simulink model "AKZO_NOBEL"  (Simulink 8.0)
settings: Solver=ode15s  StartTime=0.0  StopTime=180.0  RelTol=1e-10
PreLoadFcn:
  | k1=18.7; k2=.58; k3=.09; k4=.42; K=34.4; klA=3.3; Ks=115.83; pCO2=.9; H=737;
settings Model: Creator=David  LastModifiedBy=David
settings DataIOCC: LimitDataPoints=off  SignalLoggingSaveFormat=ModelDataLogs
settings DebuggingCC: FcnCallInpInsideContextMsg=UseLocalSettings
settings GRTTargetCC: CombineOutputUpdateFcns=off  GRTInterface=on

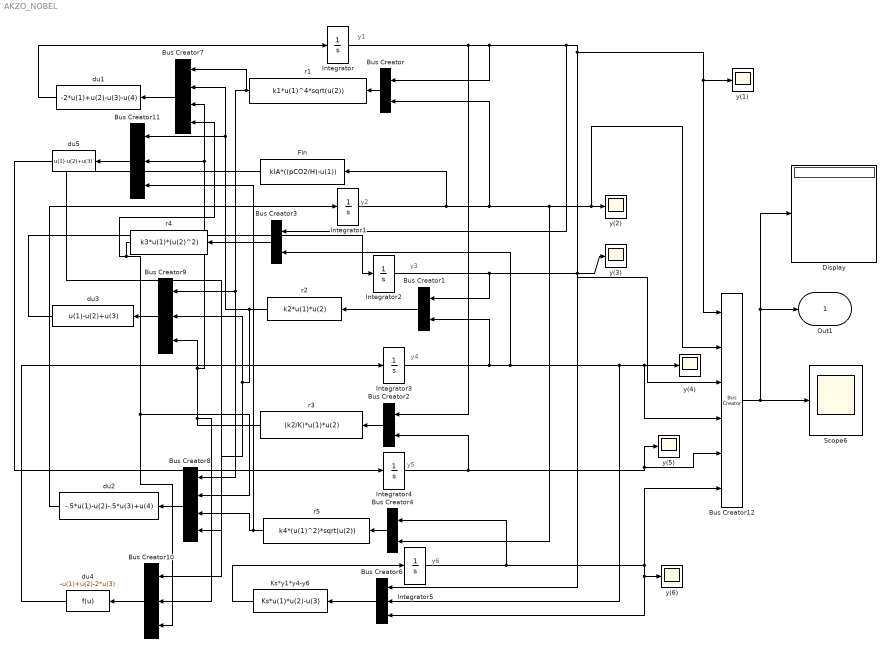
== system AKZO_NOBEL ==
  note: y1
  note: y2
  note: y3
  note: y4
  note: y5
  note: y6
  Bus Creator{,1..4} (5 alike) : BusCreator  Inputs=2
  Bus Creator{6,9..11} (4 alike) : BusCreator  Inputs=3
  Bus Creator12 : BusCreator  Inputs=6
  Bus Creator7 : BusCreator
  Bus Creator8 : BusCreator
  Display : Display
  Fin : Fcn  Expr=klA*((pCO2/H)-u(1))
  Integrator : Integrator  InitialCondition=.437
  Integrator1 : Integrator  InitialCondition=.00123
  Integrator2 : Integrator
  Integrator3 : Integrator  InitialCondition=.007
  Integrator4 : Integrator
  Integrator5 : Integrator  InitialCondition=115.83*.437*.007
  Ks*y1*y4-y6 : Fcn  Expr=Ks*u(1)*u(2)-u(3)
  Scope6 : Scope
      settings: SaveName=ScopeData6
  du1 : Fcn  Expr=-2*u(1)+u(2)-u(3)-u(4)
  du2 : Fcn  Expr=-.5*u(1)-u(2)-.5*u(3)+u(4)
  du3 : Fcn  Expr=u(1)-u(2)+u(3)
  du4 : Fcn  Expr=-u(1)+u(2)-2*u(3)
  du5 : Fcn  Expr=u(1)-u(2)+u(3)
  r1 : Fcn  Expr=k1*u(1)^4*sqrt(u(2))
  r2 : Fcn  Expr=k2*u(1)*u(2)
  r3 : Fcn  Expr=(k2/K)*u(1)*u(2)
  r4 : Fcn  Expr=k3*u(1)*(u(2)^2)
  r5 : Fcn  Expr=k4*(u(1)^2)*sqrt(u(2))
  y(1) : Scope
  y(2) : Scope
  y(3) : Scope
      settings: SaveName=ScopeData2
  y(4) : Scope
      settings: SaveName=ScopeData3
  y(5) : Scope
      settings: SaveName=ScopeData4
  y(6) : Scope
      settings: SaveName=ScopeData5
  Out1 : Outport
  wires:
  Integrator/1 -> Bus Creator/1, y(1)/1, Bus Creator12/1, Bus Creator6/1, Bus Creator3/1, Bus Creator2/1
  Integrator1/1 -> y(2)/1, Bus Creator12/2, Bus Creator4/2, Bus Creator/2, Fin/1
  Integrator2/1 -> y(3)/1, Bus Creator12/3, Bus Creator1/1
  Integrator3/1 -> y(4)/1, Bus Creator12/4, Bus Creator6/2, Bus Creator3/2, Bus Creator1/2
  Integrator4/1 -> Bus Creator2/2, y(5)/1, Bus Creator12/5
  Integrator5/1 -> Bus Creator6/3, y(6)/1, Bus Creator12/6, Bus Creator4/1
  Bus Creator/1 -> r1/1
  Bus Creator1/1 -> r2/1
  Bus Creator2/1 -> r3/1
  Bus Creator3/1 -> r4/1
  Bus Creator4/1 -> r5/1
  Bus Creator6/1 -> Ks*y1*y4-y6/1
  Ks*y1*y4-y6/1 -> Integrator5/1
  r1/1 -> Bus Creator7/1, Bus Creator8/1, Bus Creator9/1
  r2/1 -> Bus Creator9/2, Bus Creator10/1, Bus Creator7/2, Bus Creator11/1
  r3/1 -> Bus Creator9/3, Bus Creator7/3, Bus Creator11/2, Bus Creator10/2
  r4/1 -> Bus Creator7/4, Bus Creator10/3, Bus Creator8/2
  Bus Creator7/1 -> du1/1
  du1/1 -> Integrator/1
  Bus Creator8/1 -> du2/1
  r5/1 -> Bus Creator8/3, Bus Creator11/3
  Fin/1 -> Bus Creator8/4
  du2/1 -> Integrator1/1
  Bus Creator9/1 -> du3/1
  du3/1 -> Integrator2/1
  Bus Creator10/1 -> du4/1
  du4/1 -> Integrator3/1
  Bus Creator11/1 -> du5/1
  du5/1 -> Integrator4/1
  Bus Creator12/1 -> Scope6/1, Display/1, Out1/1
